simulink model "MultipleFIlterExplanation"  (R2022b)
settings: Solver=VariableStepAuto  StartTime=0.0  StopTime=inf  MaxStep=1e-3  RelTol=1e-6
libraries: commchan3 x1, dsparch4 x1
settings Model: Creator=Ceribro  LastModifiedBy=Ceribro

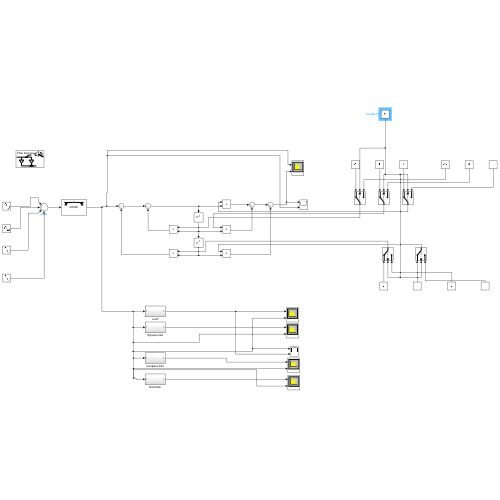
[thumbnail: Simulink's stored preview of the top-level diagram]
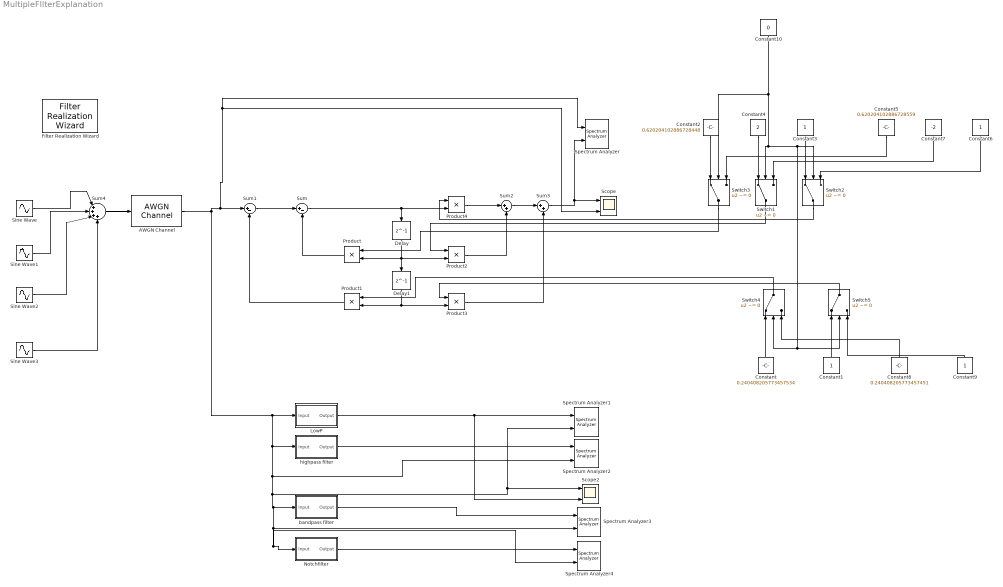
== system MultipleFIlterExplanation ==
  AWGN Channel : commchan3/AWGN Channel  InputProcessing=Columns as channels (frame based)  seed=67  noiseMode="Signal to noise ratio  (SNR)"  EbNodB=10  EsNodB=10  SNRdB=-22  bitsPerSym=1  Ps=1  Tsym=1  variance=1
  Constant : Constant  Value=0.240408205773457534
  Constant{1,3,6,9} (4 alike) : Constant
  Constant10 : Constant  Value=0
  Constant2 : Constant  Value=0.620204102886728448
  Constant4 : Constant  Value=2
  Constant5 : Constant  Value=0.620204102886728559
  Constant7 : Constant  Value=-2
  Constant8 : Constant  Value=0.240408205773457451
  Delay : Delay  DelayLength=1  InitialCondition=0
  Delay1 : Delay  DelayLength=1  InitialCondition=0
  Filter Realization Wizard : dsparch4/Filter Realization Wizard
  LowP : Subsystem  Tag=FilterWizardSubSystem
      settings: ErrorFcn=dspFilterRealizedInBasicElemsAlgLoopErrFcnCallback
  Notchfilter : Subsystem  Tag=FilterWizardSubSystem
      settings: ErrorFcn=dspFilterRealizedInBasicElemsAlgLoopErrFcnCallback
  Product{,1..4} (5 alike) : Product
  Scope : Scope  NumInputPorts=2
  Scope2 : Scope  NumInputPorts=2
  Sine Wave : Sin  Frequency=1000*2*pi  SampleTime=1/44.1e3
  Sine Wave1 : Sin  Frequency=15000*2*pi  SampleTime=1/44.1e3
  Sine Wave2 : Sin  Frequency=18000*2*pi  SampleTime=1/44.1e3
  Sine Wave3 : Sin  Frequency=7000*2*pi  SampleTime=1/44.1e3
  Spectrum Analyzer{,1..4} (5 alike) : SpectrumAnalyzer  NumInputPorts=2
  Sum : Sum  Inputs=|+-
  Sum1 : Sum  Inputs=|+-
  Sum2 : Sum  Inputs=|++
  Sum3 : Sum  Inputs=|++
  Sum4 : Sum  Inputs=|++++
  Switch{1..5} (5 alike) : Switch  Criteria=u2 ~= 0  Threshold=1  SaturateOnIntegerOverflow=off  InputSameDT=off
  bandpass filter : Subsystem  Tag=FilterWizardSubSystem
      settings: ErrorFcn=dspFilterRealizedInBasicElemsAlgLoopErrFcnCallback
  highpass filter : Subsystem  Tag=FilterWizardSubSystem
      settings: ErrorFcn=dspFilterRealizedInBasicElemsAlgLoopErrFcnCallback
  wires:
  Product4/1 -> Sum2/1
  Sum2/1 -> Sum3/1
  Sum1/1 -> Sum/1
  Delay1/1 -> Product3/2, Product1/2
  Delay/1 -> Product2/2, Product/2, Delay1/1
  Sum/1 -> Product4/2, Delay/1
  Product2/1 -> Sum2/2
  Product3/1 -> Sum3/2
  Product1/1 -> Sum1/2
  Product/1 -> Sum/2
  Sum3/1 -> Spectrum Analyzer/2, Scope/1
  Sine Wave/1 -> Sum4/1
  Sine Wave1/1 -> Sum4/2
  Sum4/1 -> AWGN Channel/1
  Sine Wave2/1 -> Sum4/3
  LowP/1(Output) -> Scope2/2, Spectrum Analyzer1/1
  Sine Wave3/1 -> Sum4/4
  AWGN Channel/1 -> Scope/2, Spectrum Analyzer/1, Sum1/1, LowP/1(Input), highpass filter/1(Input), Spectrum Analyzer2/2, Notchfilter/1(Input), Spectrum Analyzer4/2, Spectrum Analyzer3/2, bandpass filter/1(Input), Spectrum Analyzer1/2, Scope2/1
  highpass filter/1(Output) -> Spectrum Analyzer2/1
  bandpass filter/1(Output) -> Spectrum Analyzer3/1
  Notchfilter/1(Output) -> Spectrum Analyzer4/1
  Constant2/1 -> Switch3/1
  Switch3/1 -> Product/1
  Constant4/1 -> Switch1/1
  Switch1/1 -> Product2/1
  Constant3/1 -> Switch2/1
  Switch2/1 -> Product4/1
  Constant/1 -> Switch4/1
  Switch4/1 -> Product1/1
  Constant1/1 -> Switch5/1
  Switch5/1 -> Product3/1
  Constant5/1 -> Switch3/3
  Constant7/1 -> Switch1/3
  Constant6/1 -> Switch2/3
  Constant8/1 -> Switch4/3
  Constant9/1 -> Switch5/3
  Constant10/1 -> Switch4/2, Switch5/2, Switch2/2, Switch1/2, Switch3/2

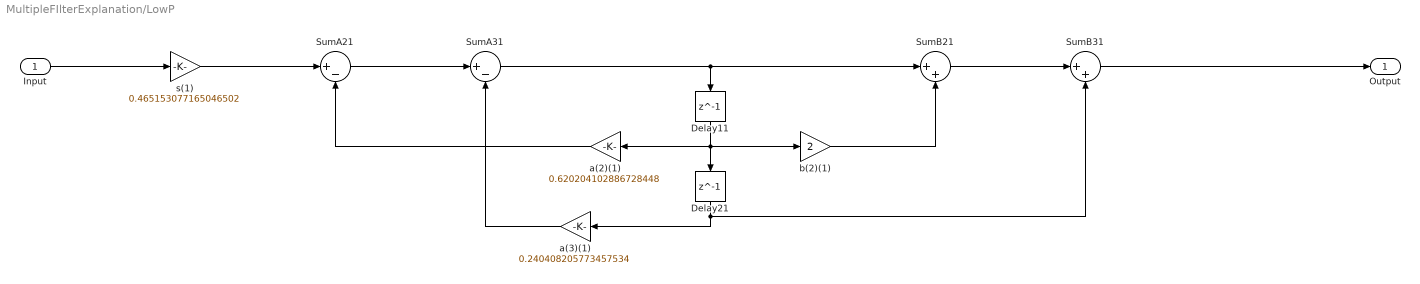
== system MultipleFIlterExplanation/LowP ==
  Input : Inport
  Delay11 : Delay  DelayLength=1  InitialCondition=0
  Delay21 : Delay  DelayLength=1  InitialCondition=0
  SumA21 : Sum  Inputs=|+-  RndMeth=Nearest  SaturateOnIntegerOverflow=on  OutDataTypeStr=Inherit: Same as first input
  SumA31 : Sum  Inputs=|+-  RndMeth=Nearest  SaturateOnIntegerOverflow=on  OutDataTypeStr=Inherit: Same as first input
  SumB21 : Sum  Inputs=|++  RndMeth=Nearest  SaturateOnIntegerOverflow=on  OutDataTypeStr=Inherit: Same as first input
  SumB31 : Sum  Inputs=|++  RndMeth=Nearest  SaturateOnIntegerOverflow=on  OutDataTypeStr=Inherit: Same as first input
  a(2)(1) : Gain  Gain=0.620204102886728448  ParamDataTypeStr=double  RndMeth=Nearest  SaturateOnIntegerOverflow=on  OutDataTypeStr=Inherit: Same as input
  a(3)(1) : Gain  Gain=0.240408205773457534  ParamDataTypeStr=double  RndMeth=Nearest  SaturateOnIntegerOverflow=on  OutDataTypeStr=Inherit: Same as input
  b(2)(1) : Gain  Gain=2  ParamDataTypeStr=double  RndMeth=Nearest  SaturateOnIntegerOverflow=on  OutDataTypeStr=Inherit: Same as input
  s(1) : Gain  Gain=0.465153077165046502  ParamDataTypeStr=double  RndMeth=Nearest  SaturateOnIntegerOverflow=on  OutDataTypeStr=Inherit: Same as input
  Output : Outport
  wires:
  Input/1 -> s(1)/1
  s(1)/1 -> SumA21/1
  SumA21/1 -> SumA31/1
  SumA31/1 -> SumB21/1, Delay11/1
  SumB21/1 -> SumB31/1
  SumB31/1 -> Output/1
  a(2)(1)/1 -> SumA21/2
  Delay11/1 -> a(2)(1)/1, b(2)(1)/1, Delay21/1
  b(2)(1)/1 -> SumB21/2
  a(3)(1)/1 -> SumA31/2
  Delay21/1 -> a(3)(1)/1, SumB31/2

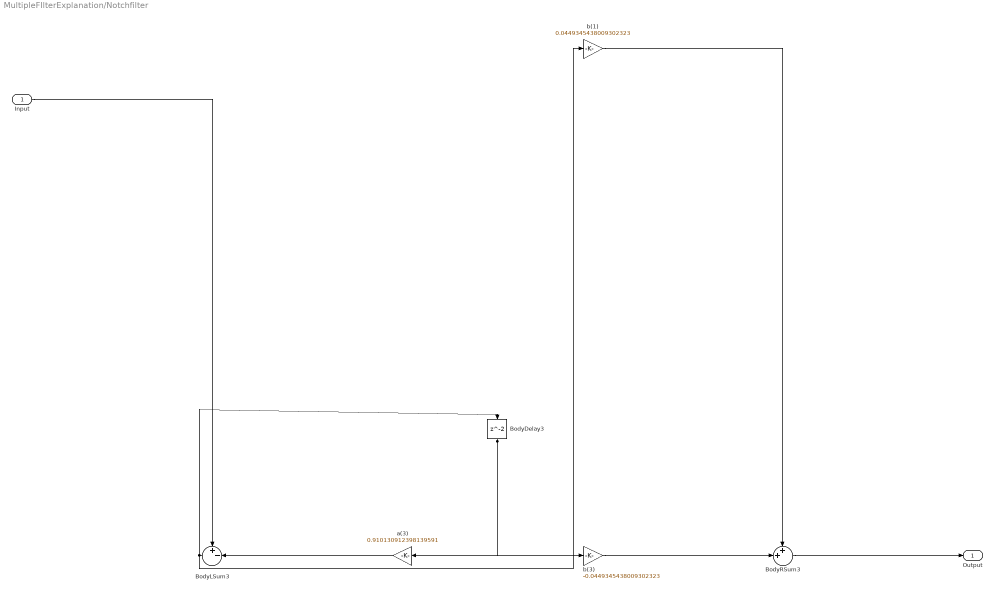
== system MultipleFIlterExplanation/Notchfilter ==
  Input : Inport
  BodyDelay3 : Delay  InitialCondition=0
  BodyLSum3 : Sum  Inputs=+-|  RndMeth=Nearest  SaturateOnIntegerOverflow=on  OutDataTypeStr=Inherit: Same as first input
  BodyRSum3 : Sum  Inputs=++|  RndMeth=Nearest  SaturateOnIntegerOverflow=on  OutDataTypeStr=Inherit: Same as first input
  a(3) : Gain  Gain=0.910130912398139591  ParamDataTypeStr=double  RndMeth=Nearest  SaturateOnIntegerOverflow=on  OutDataTypeStr=Inherit: Same as input
  b(1) : Gain  Gain=0.0449345438009302323  ParamDataTypeStr=double  RndMeth=Nearest  SaturateOnIntegerOverflow=on  OutDataTypeStr=Inherit: Same as input
  b(3) : Gain  Gain=-0.0449345438009302323  ParamDataTypeStr=double  RndMeth=Nearest  SaturateOnIntegerOverflow=on  OutDataTypeStr=Inherit: Same as input
  Output : Outport
  wires:
  b(1)/1 -> BodyRSum3/1
  Input/1 -> BodyLSum3/1
  BodyLSum3/1 -> b(1)/1, BodyDelay3/1
  a(3)/1 -> BodyLSum3/2
  BodyDelay3/1 -> a(3)/1, b(3)/1
  b(3)/1 -> BodyRSum3/2
  BodyRSum3/1 -> Output/1

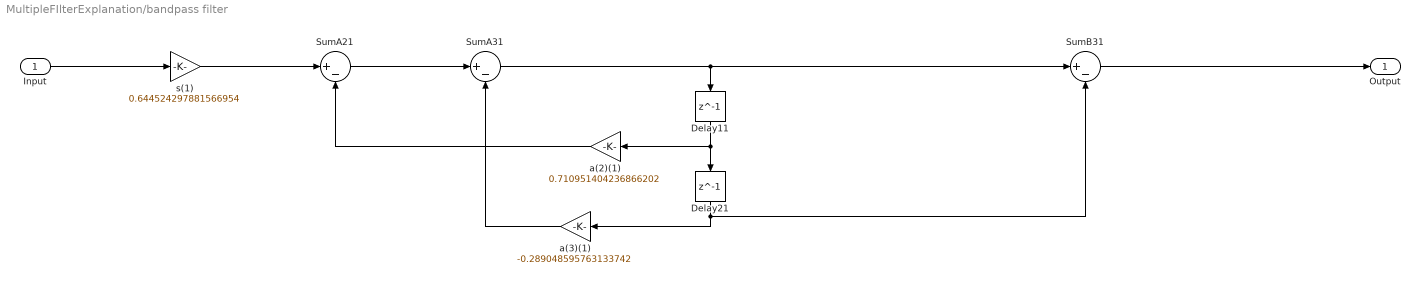
== system MultipleFIlterExplanation/bandpass filter ==
  Input : Inport
  Delay11 : Delay  DelayLength=1  InitialCondition=0
  Delay21 : Delay  DelayLength=1  InitialCondition=0
  SumA21 : Sum  Inputs=|+-  RndMeth=Nearest  SaturateOnIntegerOverflow=on  OutDataTypeStr=Inherit: Same as first input
  SumA31 : Sum  Inputs=|+-  RndMeth=Nearest  SaturateOnIntegerOverflow=on  OutDataTypeStr=Inherit: Same as first input
  SumB31 : Sum  Inputs=|+-  RndMeth=Nearest  SaturateOnIntegerOverflow=on  OutDataTypeStr=Inherit: Same as first input
  a(2)(1) : Gain  Gain=0.710951404236866202  ParamDataTypeStr=double  RndMeth=Nearest  SaturateOnIntegerOverflow=on  OutDataTypeStr=Inherit: Same as input
  a(3)(1) : Gain  Gain=-0.289048595763133742  ParamDataTypeStr=double  RndMeth=Nearest  SaturateOnIntegerOverflow=on  OutDataTypeStr=Inherit: Same as input
  s(1) : Gain  Gain=0.644524297881566954  ParamDataTypeStr=double  RndMeth=Nearest  SaturateOnIntegerOverflow=on  OutDataTypeStr=Inherit: Same as input
  Output : Outport
  wires:
  Input/1 -> s(1)/1
  s(1)/1 -> SumA21/1
  SumA21/1 -> SumA31/1
  SumA31/1 -> SumB31/1, Delay11/1
  SumB31/1 -> Output/1
  a(2)(1)/1 -> SumA21/2
  Delay11/1 -> a(2)(1)/1, Delay21/1
  a(3)(1)/1 -> SumA31/2
  Delay21/1 -> a(3)(1)/1, SumB31/2

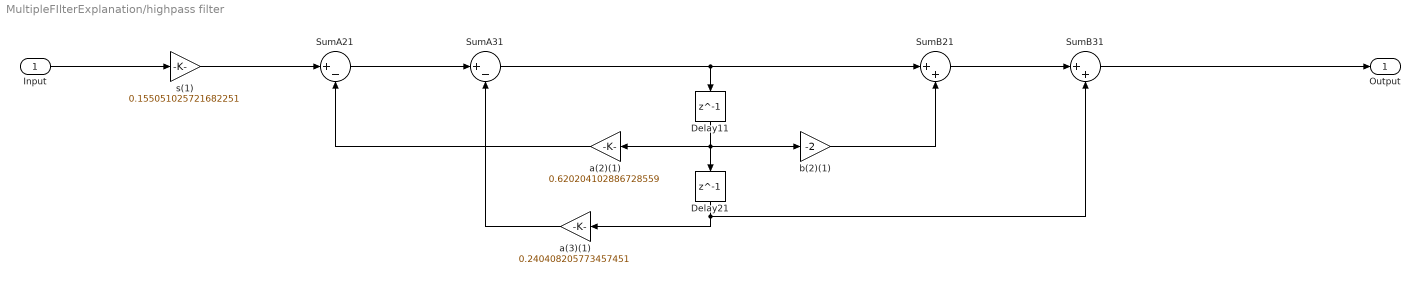
== system MultipleFIlterExplanation/highpass filter ==
  Input : Inport
  Delay11 : Delay  DelayLength=1  InitialCondition=0
  Delay21 : Delay  DelayLength=1  InitialCondition=0
  SumA21 : Sum  Inputs=|+-  RndMeth=Nearest  SaturateOnIntegerOverflow=on  OutDataTypeStr=Inherit: Same as first input
  SumA31 : Sum  Inputs=|+-  RndMeth=Nearest  SaturateOnIntegerOverflow=on  OutDataTypeStr=Inherit: Same as first input
  SumB21 : Sum  Inputs=|++  RndMeth=Nearest  SaturateOnIntegerOverflow=on  OutDataTypeStr=Inherit: Same as first input
  SumB31 : Sum  Inputs=|++  RndMeth=Nearest  SaturateOnIntegerOverflow=on  OutDataTypeStr=Inherit: Same as first input
  a(2)(1) : Gain  Gain=0.620204102886728559  ParamDataTypeStr=double  RndMeth=Nearest  SaturateOnIntegerOverflow=on  OutDataTypeStr=Inherit: Same as input
  a(3)(1) : Gain  Gain=0.240408205773457451  ParamDataTypeStr=double  RndMeth=Nearest  SaturateOnIntegerOverflow=on  OutDataTypeStr=Inherit: Same as input
  b(2)(1) : Gain  Gain=-2  ParamDataTypeStr=double  RndMeth=Nearest  SaturateOnIntegerOverflow=on  OutDataTypeStr=Inherit: Same as input
  s(1) : Gain  Gain=0.155051025721682251  ParamDataTypeStr=double  RndMeth=Nearest  SaturateOnIntegerOverflow=on  OutDataTypeStr=Inherit: Same as input
  Output : Outport
  wires:
  Input/1 -> s(1)/1
  s(1)/1 -> SumA21/1
  SumA21/1 -> SumA31/1
  SumA31/1 -> SumB21/1, Delay11/1
  SumB21/1 -> SumB31/1
  SumB31/1 -> Output/1
  a(2)(1)/1 -> SumA21/2
  Delay11/1 -> a(2)(1)/1, b(2)(1)/1, Delay21/1
  b(2)(1)/1 -> SumB21/2
  a(3)(1)/1 -> SumA31/2
  Delay21/1 -> a(3)(1)/1, SumB31/2
